simulink model "PID tuning with different Methods"  (R2021b)
settings: Solver=VariableStepAuto  StartTime=0.0  StopTime=30  RelTol=1e-3
settings Model: Creator=mahya  LastModifiedBy=mahya

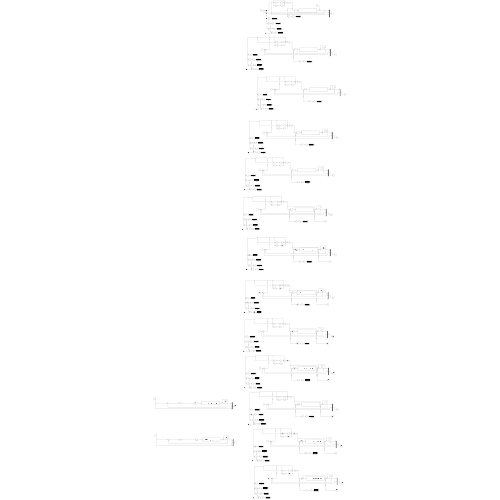
[thumbnail: Simulink's stored preview of the top-level diagram]
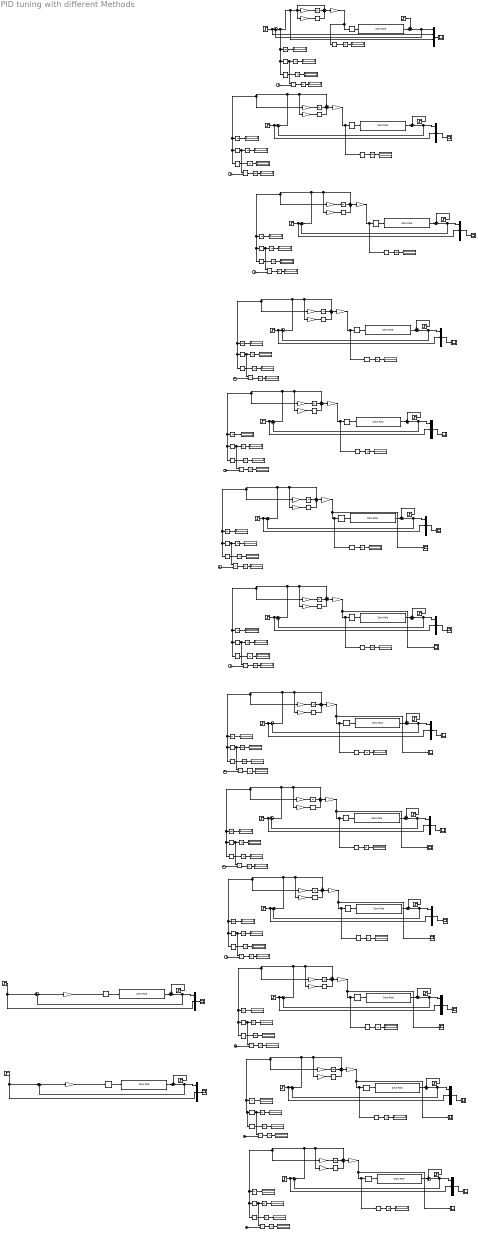
== system PID tuning with different Methods ==
  1/Ti : Gain  Gain=1/1.5
  1/Ti10 : Gain  Gain=1/1.7225
  1/Ti11 : Gain  Gain=1/1.4
  1/Ti12 : Gain  Gain=1/0.83
  1/Ti13 : Gain  Gain=0.7
  1/Ti2 : Gain  Gain=1/1.397
  1/Ti3 : Gain  Gain=1/2.66
  1/Ti4 : Gain  Gain=1/1.9
  1/Ti5 : Gain  Gain=1/1.8
  1/Ti6 : Gain  Gain=1/1.5
  1/Ti7 : Gain  Gain=1/1.378
  1/Ti8 : Gain  Gain=1/1.272
  1/Ti9 : Gain  Gain=1/2.385
  Abs{,2..26} (26 alike) : Abs
  Clock{,2..13} (13 alike) : Clock
  Derivative{,2..13} (13 alike) : Derivative
  IAE{,2..13} (13 alike) : Display
  IAE control sig{,1..12} (13 alike) : Display
  IE{,2..13} (13 alike) : Display
  ISE{,2..13} (13 alike) : Display
  ITAE{,2..13} (13 alike) : Display
  Integrator{,2..6,11..82} (78 alike) : Integrator
  Kp : Gain  Gain=1.05
  Kp10 : Gain  Gain=0.75
  Kp11 : Gain  Gain=0.72
  Kp12 : Gain  Gain=1.2
  Kp13 : Gain  Gain=0.98
  Kp14 : Gain  Gain=0.9
  Kp15 : Gain  Gain=0.7
  Kp2 : Gain  Gain=0.897
  Kp3 : Gain  Gain=1.2
  Kp4 : Gain  Gain=0.76
  Kp5 : Gain  Gain=0.76
  Kp6 : Gain  Gain=1.52
  Kp7 : Gain  Gain=0.65
  Kp8 : Gain  Gain=0.9
  Kp9 : Gain  Gain=0.45
  Math Function{,2..13} (13 alike) : Math  Operator=square  SaturateOnIntegerOverflow=on
  Mux{3..16} (14 alike) : Mux  Inputs=3
  Mux2 : Mux
  Product{,2..13} (13 alike) : Product
  Scope{2..24} (23 alike) : Scope
  Step{4,6,8,10,12,14,16,18,20,22,26,28,30,32} (14 alike) : Step  Time=0  SampleTime=0
  Step{5,7,9,11,13,15,17,19,21,23,25,27,29,31,33} (15 alike) : Step  Time=15  After=0.5  SampleTime=0
  Step24 : Step  Time=0  After=0  SampleTime=0
  Sum{1,8,12,15,18,21,24,27,30,33,36,41,46} (13 alike) : Sum  Inputs=+++
  Sum{7,10..11,14,17,20,23,26,29,32,35,39..40,44..45} (15 alike) : Sum  Inputs=|+-
  Sum{6,9,13,16,19,22,25,28,31,34,37..38,42..43,47} (15 alike) : Sum  Inputs=++|
  Td : Gain  Gain=0.375
  Td10 : Gain  Gain=0
  Td11 : Gain  Gain=0.35
  Td12 : Gain  Gain=0.333
  Td13 : Gain  Gain=0.2
  Td2 : Gain  Gain=0.248
  Td3 : Gain  Gain=0.3525
  Td4 : Gain  Gain=0.375
  Td5 : Gain  Gain=0.315
  Td6 : Gain  Gain=0.315
  Td7 : Gain  Gain=0.715
  Td8 : Gain  Gain=0.715
  Td9 : Gain  Gain=0.106
  Transport Delay{2..16} (15 alike) : TransportDelay  DelayTime=0.633
  Zero-Pole{2..16} (15 alike) : ZeroPole  Zeros=[]  Poles=[-1 -5 -25 -125]  Gain=[2*15625]
  wires:
  Sum7/1 -> Mux2/3, Td/1, 1/Ti/1, Sum1/1, Math Function/1, Abs/1, Integrator3/1
  Td/1 -> Derivative/1
  Integrator/1 -> Sum1/2
  Derivative/1 -> Sum1/3
  Sum1/1 -> Kp/1
  1/Ti/1 -> Integrator/1
  Step4/1 -> Sum7/1, Mux2/2
  Sum6/1 -> Mux2/1, Sum7/2
  Step5/1 -> Sum6/1
  Zero-Pole2/1 -> Sum6/2
  Transport Delay2/1 -> Zero-Pole2/1
  Mux2/1 -> Scope2/1
  Kp/1 -> Abs3/1, Transport Delay2/1
  Zero-Pole3/1 -> Sum9/2
  Sum9/1 -> Mux3/1, Sum10/2
  Mux3/1 -> Scope3/1
  Transport Delay3/1 -> Zero-Pole3/1
  Step6/1 -> Sum10/1, Mux3/2
  Kp2/1 -> Abs4/1, Transport Delay3/1
  Integrator2/1 -> Sum8/2
  Td2/1 -> Derivative2/1
  1/Ti2/1 -> Integrator2/1
  Step7/1 -> Sum9/1
  Derivative2/1 -> Sum8/3
  Sum8/1 -> Kp2/1
  Integrator3/1 -> IE/1
  Abs/1 -> Product/1, Integrator4/1
  Integrator4/1 -> IAE/1
  Integrator5/1 -> ISE/1
  Math Function/1 -> Integrator5/1
  Clock/1 -> Product/2
  Integrator6/1 -> ITAE/1
  Product/1 -> Integrator6/1
  Integrator14/1 -> ISE2/1
  Clock2/1 -> Product2/2
  Sum10/1 -> Td2/1, Sum8/1, Math Function2/1, Abs2/1, Integrator12/1, 1/Ti2/1
  Integrator11/1 -> ITAE2/1
  Integrator13/1 -> IAE2/1
  Abs2/1 -> Product2/1, Integrator13/1
  Math Function2/1 -> Integrator14/1
  Integrator12/1 -> IE2/1
  Product2/1 -> Integrator11/1
  Integrator15/1 -> IAE control sig/1
  Abs3/1 -> Integrator15/1
  Integrator16/1 -> IAE control sig1/1
  Abs4/1 -> Integrator16/1
  Integrator21/1 -> IAE control sig2/1
  Abs6/1 -> Integrator21/1
  Abs5/1 -> Product3/1, Integrator19/1
  Integrator19/1 -> IAE3/1
  Integrator17/1 -> ITAE3/1
  Sum11/1 -> Td3/1, Sum12/1, Math Function3/1, Abs5/1, Integrator18/1, 1/Ti3/1
  Kp3/1 -> Abs6/1, Transport Delay4/1
  Sum12/1 -> Kp3/1
  1/Ti3/1 -> Integrator22/1
  Td3/1 -> Derivative3/1
  Step9/1 -> Sum13/1
  Integrator22/1 -> Sum12/2
  Mux4/1 -> Scope4/1
  Derivative3/1 -> Sum12/3
  Zero-Pole4/1 -> Sum13/2
  Sum13/1 -> Mux4/1, Sum11/2
  Transport Delay4/1 -> Zero-Pole4/1
  Integrator20/1 -> ISE3/1
  Step8/1 -> Sum11/1, Mux4/2
  Clock3/1 -> Product3/2
  Product3/1 -> Integrator17/1
  Integrator18/1 -> IE3/1
  Math Function3/1 -> Integrator20/1
  Math Function4/1 -> Integrator26/1
  Integrator24/1 -> IE4/1
  Sum16/1 -> Mux5/1, Sum14/2
  Integrator26/1 -> ISE4/1
  Step10/1 -> Sum14/1, Mux5/2
  Clock4/1 -> Product4/2
  Product4/1 -> Integrator23/1
  Transport Delay5/1 -> Zero-Pole5/1
  Td4/1 -> Derivative4/1
  1/Ti4/1 -> Integrator28/1
  Derivative4/1 -> Sum15/3
  Sum15/1 -> Kp4/1
  Integrator28/1 -> Sum15/2
  Mux5/1 -> Scope5/1
  Step11/1 -> Sum16/1
  Kp4/1 -> Abs8/1, Transport Delay5/1
  Integrator23/1 -> ITAE4/1
  Integrator25/1 -> IAE4/1
  Zero-Pole5/1 -> Sum16/2
  Abs7/1 -> Product4/1, Integrator25/1
  Sum14/1 -> Td4/1, Sum15/1, Math Function4/1, Abs7/1, Integrator24/1, 1/Ti4/1
  Abs8/1 -> Integrator27/1
  Integrator27/1 -> IAE control sig3/1
  Abs10/1 -> Integrator33/1
  Sum17/1 -> Td5/1, Sum18/1, Math Function5/1, Abs9/1, Integrator30/1, 1/Ti5/1
  Integrator29/1 -> ITAE5/1
  Kp5/1 -> Abs10/1, Transport Delay6/1
  Zero-Pole6/1 -> Sum19/2
  Abs9/1 -> Product5/1, Integrator31/1
  Integrator34/1 -> Sum18/2
  1/Ti5/1 -> Integrator34/1
  Sum18/1 -> Kp5/1
  Product5/1 -> Integrator29/1
  Integrator31/1 -> IAE5/1
  Mux6/1 -> Scope6/1
  Step13/1 -> Sum19/1
  Td5/1 -> Derivative5/1
  Derivative5/1 -> Sum18/3
  Transport Delay6/1 -> Zero-Pole6/1
  Sum19/1 -> Mux6/1, Sum17/2
  Step12/1 -> Sum17/1, Mux6/2
  Integrator32/1 -> ISE5/1
  Clock5/1 -> Product5/2
  Integrator30/1 -> IE5/1
  Math Function5/1 -> Integrator32/1
  Integrator33/1 -> IAE control sig4/1
  Abs12/1 -> Integrator39/1
  Sum20/1 -> Td6/1, Sum21/1, Math Function6/1, Abs11/1, Integrator36/1, 1/Ti6/1
  Integrator35/1 -> ITAE6/1
  Zero-Pole7/1 -> Sum22/2
  Abs11/1 -> Product6/1, Integrator37/1
  Integrator40/1 -> Sum21/2
  1/Ti6/1 -> Integrator40/1
  Sum21/1 -> Kp6/1
  Product6/1 -> Integrator35/1
  Integrator37/1 -> IAE6/1
  Mux7/1 -> Scope7/1
  Step15/1 -> Sum22/1
  Td6/1 -> Derivative6/1
  Derivative6/1 -> Sum21/3
  Transport Delay7/1 -> Zero-Pole7/1
  Sum22/1 -> Mux7/1, Sum20/2
  Step14/1 -> Sum20/1, Mux7/2
  Integrator38/1 -> ISE6/1
  Clock6/1 -> Product6/2
  Integrator36/1 -> IE6/1
  Math Function6/1 -> Integrator38/1
  Integrator39/1 -> IAE control sig5/1
  Kp6/1 -> Scope8/1, Abs12/1, Transport Delay7/1
  Math Function7/1 -> Integrator44/1
  Integrator45/1 -> IAE control sig6/1
  Integrator42/1 -> IE7/1
  Clock7/1 -> Product7/2
  Integrator44/1 -> ISE7/1
  Transport Delay8/1 -> Zero-Pole8/1
  Step16/1 -> Sum23/1, Mux8/2
  Product7/1 -> Integrator41/1
  Integrator46/1 -> Sum24/2
  Derivative7/1 -> Sum24/3
  Sum24/1 -> Kp7/1
  1/Ti7/1 -> Integrator46/1
  Zero-Pole8/1 -> Sum25/2
  Abs13/1 -> Product7/1, Integrator43/1
  Kp7/1 -> Scope10/1, Abs14/1, Transport Delay8/1
  Integrator41/1 -> ITAE7/1
  Step17/1 -> Sum25/1
  Mux8/1 -> Scope9/1
  Sum23/1 -> Td7/1, Sum24/1, Math Function7/1, Abs13/1, Integrator42/1, 1/Ti7/1
  Abs14/1 -> Integrator45/1
  Sum25/1 -> Mux8/1, Sum23/2
  Td7/1 -> Derivative7/1
  Integrator43/1 -> IAE7/1
  Abs16/1 -> Integrator51/1
  Integrator49/1 -> IAE8/1
  Td8/1 -> Derivative8/1
  Sum28/1 -> Mux9/1, Sum26/2
  Abs15/1 -> Product8/1, Integrator49/1
  Mux9/1 -> Scope12/1
  Kp8/1 -> Scope11/1, Abs16/1, Transport Delay9/1
  Step19/1 -> Sum28/1
  Integrator47/1 -> ITAE8/1
  1/Ti8/1 -> Integrator52/1
  Zero-Pole9/1 -> Sum28/2
  Integrator52/1 -> Sum27/2
  Derivative8/1 -> Sum27/3
  Sum27/1 -> Kp8/1
  Sum26/1 -> Td8/1, Sum27/1, Math Function8/1, Abs15/1, Integrator48/1, 1/Ti8/1
  Step18/1 -> Sum26/1, Mux9/2
  Transport Delay9/1 -> Zero-Pole9/1
  Integrator50/1 -> ISE8/1
  Clock8/1 -> Product8/2
  Math Function8/1 -> Integrator50/1
  Product8/1 -> Integrator47/1
  Integrator48/1 -> IE8/1
  Integrator51/1 -> IAE control sig7/1
  Integrator57/1 -> IAE control sig8/1
  Math Function9/1 -> Integrator56/1
  Clock9/1 -> Product9/2
  Integrator56/1 -> ISE9/1
  Transport Delay10/1 -> Zero-Pole10/1
  Integrator54/1 -> IE9/1
  Step21/1 -> Sum31/1
  Kp9/1 -> Scope13/1, Abs18/1, Transport Delay10/1
  Product9/1 -> Integrator53/1
  Mux10/1 -> Scope14/1
  Step20/1 -> Sum29/1, Mux10/2
  Abs17/1 -> Product9/1, Integrator55/1
  Integrator55/1 -> IAE9/1
  Td9/1 -> Derivative9/1
  Integrator53/1 -> ITAE9/1
  Sum30/1 -> Kp9/1
  Integrator58/1 -> Sum30/2
  1/Ti9/1 -> Integrator58/1
  Zero-Pole10/1 -> Sum31/2
  Abs18/1 -> Integrator57/1
  Sum29/1 -> Td9/1, Sum30/1, Math Function9/1, Abs17/1, Integrator54/1, 1/Ti9/1
  Derivative9/1 -> Sum30/3
  Sum31/1 -> Mux10/1, Sum29/2
  Derivative10/1 -> Sum33/3
  Sum32/1 -> Td10/1, Sum33/1, Math Function10/1, Abs19/1, Integrator60/1, 1/Ti10/1
  Abs20/1 -> Integrator63/1
  Td10/1 -> Derivative10/1
  1/Ti10/1 -> Integrator64/1
  Integrator59/1 -> ITAE10/1
  Integrator61/1 -> IAE10/1
  Zero-Pole11/1 -> Sum34/2
  Integrator64/1 -> Sum33/2
  Sum33/1 -> Kp10/1
  Abs19/1 -> Product10/1, Integrator61/1
  Step22/1 -> Sum32/1, Mux11/2
  Product10/1 -> Integrator59/1
  Sum34/1 -> Mux11/1, Sum32/2
  Kp10/1 -> Scope15/1, Abs20/1, Transport Delay11/1
  Step23/1 -> Sum34/1
  Integrator60/1 -> IE10/1
  Mux11/1 -> Scope16/1
  Integrator62/1 -> ISE10/1
  Transport Delay11/1 -> Zero-Pole11/1
  Clock10/1 -> Product10/2
  Math Function10/1 -> Integrator62/1
  Integrator63/1 -> IAE control sig9/1
  Sum35/1 -> Td11/1, Sum36/1, Math Function11/1, Abs21/1, Integrator66/1, 1/Ti11/1
  Derivative11/1 -> Sum36/3
  Sum36/1 -> Kp11/1
  Integrator70/1 -> Sum36/2
  Integrator67/1 -> IAE11/1
  Abs22/1 -> Integrator69/1
  Integrator65/1 -> ITAE11/1
  Td11/1 -> Derivative11/1
  1/Ti11/1 -> Integrator70/1
  Math Function11/1 -> Integrator68/1
  Integrator69/1 -> IAE control sig10/1
  Clock11/1 -> Product11/2
  Transport Delay12/1 -> Zero-Pole12/1
  Kp11/1 -> Scope17/1, Abs22/1, Transport Delay12/1
  Integrator66/1 -> IE11/1
  Step25/1 -> Sum37/1
  Step24/1 -> Sum35/1, Mux12/2
  Sum37/1 -> Mux12/1, Sum35/2
  Integrator68/1 -> ISE11/1
  Product11/1 -> Integrator65/1
  Zero-Pole12/1 -> Sum37/2
  Abs21/1 -> Product11/1, Integrator67/1
  Mux12/1 -> Scope18/1
  Step27/1 -> Sum38/1
  Step26/1 -> Mux13/2, Sum39/1
  Transport Delay13/1 -> Zero-Pole13/1
  Sum39/1 -> Kp12/1
  Sum38/1 -> Mux13/1, Sum39/2
  Zero-Pole13/1 -> Sum38/2
  Mux13/1 -> Scope19/1
  Kp12/1 -> Transport Delay13/1
  Transport Delay14/1 -> Zero-Pole14/1
  Clock12/1 -> Product12/2
  Integrator75/1 -> IAE control sig11/1
  Math Function12/1 -> Integrator74/1
  Mux14/1 -> Scope21/1
  Product12/1 -> Integrator71/1
  Zero-Pole14/1 -> Sum42/2
  Sum42/1 -> Mux14/1, Sum40/2
  Integrator74/1 -> ISE12/1
  Integrator72/1 -> IE12/1
  Kp13/1 -> Scope20/1, Abs24/1, Transport Delay14/1
  1/Ti12/1 -> Integrator76/1
  Td12/1 -> Derivative12/1
  Integrator71/1 -> ITAE12/1
  Integrator73/1 -> IAE12/1
  Sum41/1 -> Kp13/1
  Abs24/1 -> Integrator75/1
  Abs23/1 -> Product12/1, Integrator73/1
  Integrator76/1 -> Sum41/2
  Derivative12/1 -> Sum41/3
  Step29/1 -> Sum42/1
  Sum40/1 -> Td12/1, Sum41/1, Math Function12/1, Abs23/1, Integrator72/1, 1/Ti12/1
  Step28/1 -> Sum40/1, Mux14/2
  Kp14/1 -> Transport Delay15/1
  Mux15/1 -> Scope22/1
  Zero-Pole15/1 -> Sum43/2
  Sum43/1 -> Mux15/1, Sum44/2
  Sum44/1 -> Kp14/1
  Transport Delay15/1 -> Zero-Pole15/1
  Step30/1 -> Mux15/2, Sum44/1
  Step31/1 -> Sum43/1
  Step32/1 -> Sum45/1, Mux16/2
  Sum45/1 -> Td13/1, Sum46/1, Math Function13/1, Abs25/1, Integrator78/1, 1/Ti13/1
  Step33/1 -> Sum47/1
  Math Function13/1 -> Integrator80/1
  Integrator81/1 -> IAE control sig12/1
  Clock13/1 -> Product13/2
  Sum47/1 -> Mux16/1, Sum45/2
  Zero-Pole16/1 -> Sum47/2
  Product13/1 -> Integrator77/1
  Mux16/1 -> Scope24/1
  Integrator78/1 -> IE13/1
  Integrator80/1 -> ISE13/1
  Abs26/1 -> Integrator81/1
  Transport Delay16/1 -> Zero-Pole16/1
  Td13/1 -> Derivative13/1
  Integrator82/1 -> Sum46/2
  Integrator79/1 -> IAE13/1
  1/Ti13/1 -> Integrator82/1
  Sum46/1 -> Kp15/1
  Abs25/1 -> Product13/1, Integrator79/1
  Kp15/1 -> Scope23/1, Abs26/1, Transport Delay16/1
  Derivative13/1 -> Sum46/3
  Integrator77/1 -> ITAE13/1
